simulink model "PCCI_Motor"  (R2023b)
settings: Solver=FixedStepDiscrete  StartTime=0.0  StopTime=10  FixedStep=0.01  RelTol=1e-3
settings Model: Creator=LENOVO-MCC  LastModifiedBy=LENOVO-MCC
settings OptimizationCC: DefaultParameterBehavior=Inlined  EnhancedBackFolding=on  PassReuseOutputArgsAs=Individual arguments  ZeroExternalMemoryAtStartup=off  ZeroInternalMemoryAtStartup=off  OptimizeBlockOrder=speed  DifferentSizesBufferReuse=on  OptimizationCustomize=off  EfficientTunableParamExpr=on
settings DebuggingCC: ParameterTunabilityLossMsg=error
settings SFSimCC: MATLABDynamicMemAlloc=off
settings RTWCC: Description=Embedded Coder  SystemTargetFile=ert.tlc  GenCodeOnly=on  TemplateMakefile=ert_default_tmf  GenerateReport=on  LaunchReport=on  GenerateCodeMetricsReport=on
settings CodeAppCC: ForceParamTrailComments=on  IgnoreCustomStorageClasses=off  OperatorAnnotations=on  SimulinkDataObjDesc=on  SFDataObjDesc=on  InsertBlockDesc=on
settings ERTTargetCC: TargetLangStandard=C99 (ISO)  GenerateSampleERTMain=on  InlinedParameterPlacement=NonHierarchical  ERTCustomFileTemplate=example_file_process.tlc

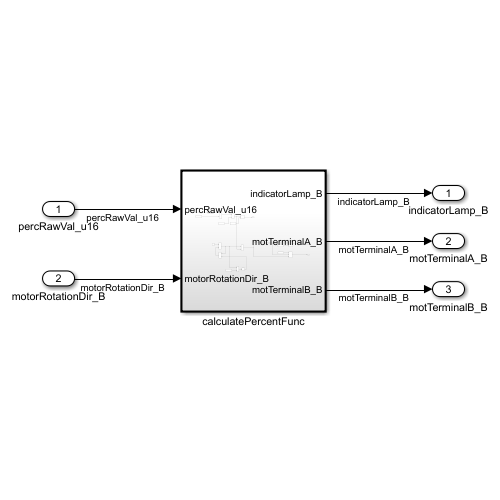
[thumbnail: Simulink's stored preview of the top-level diagram]
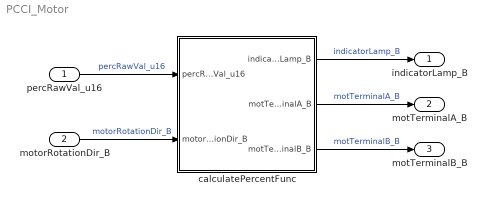
== system PCCI_Motor ==
  percRawVal_u16 : Inport  OutDataTypeStr=uint16
  motorRotationDir_B : Inport  Port=2  OutDataTypeStr=boolean
  calculatePercentFunc : Subsystem  TreatAsAtomicUnit=on
      settings: RTWFcnNameOpts=Use subsystem name  RTWFileNameOpts=Use subsystem name
  indicatorLamp_B : Outport  OutDataTypeStr=boolean
  motTerminalA_B : Outport  Port=2  OutDataTypeStr=boolean
  motTerminalB_B : Outport  Port=3  OutDataTypeStr=boolean
  wires:
  calculatePercentFunc/1(indicatorLamp_B) -> indicatorLamp_B/1  "indicatorLamp_B"
  percRawVal_u16/1 -> calculatePercentFunc/1(percRawVal_u16)  "percRawVal_u16"
  calculatePercentFunc/2(motTerminalA_B) -> motTerminalA_B/1  "motTerminalA_B"
  calculatePercentFunc/3(motTerminalB_B) -> motTerminalB_B/1  "motTerminalB_B"
  motorRotationDir_B/1 -> calculatePercentFunc/2(motorRotationDir_B)  "motorRotationDir_B"

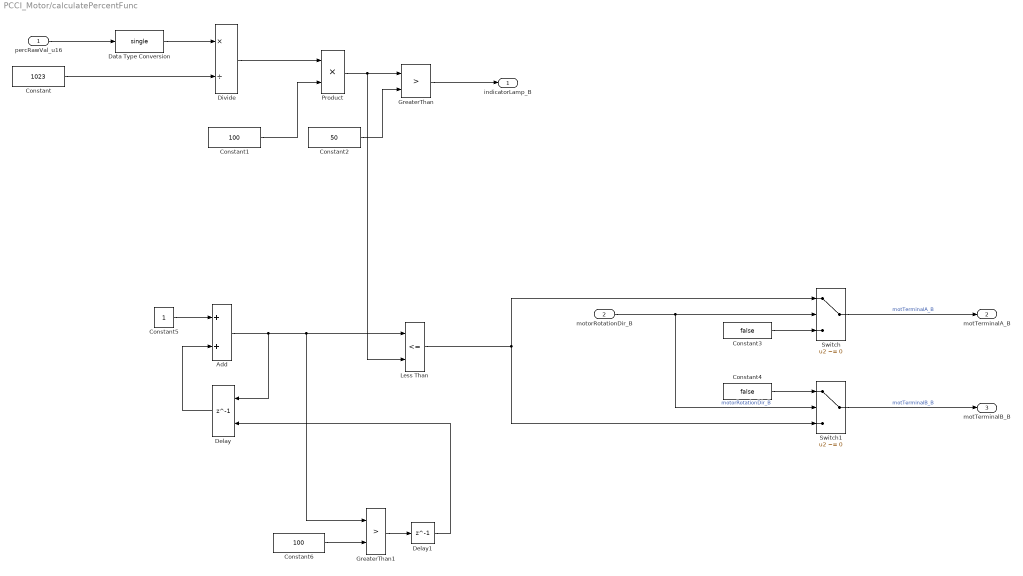
== system PCCI_Motor/calculatePercentFunc ==
  percRawVal_u16 : Inport  OutDataTypeStr=uint16
  motorRotationDir_B : Inport  Port=2  OutDataTypeStr=boolean
  Add : Sum
  Constant : Constant  Value=1023  OutDataTypeStr=single
  Constant1 : Constant  Value=100  OutDataTypeStr=int8
  Constant2 : Constant  Value=50  OutDataTypeStr=int8
  Constant3 : Constant  Value=false  OutDataTypeStr=boolean
  Constant4 : Constant  Value=false  OutDataTypeStr=boolean
  Constant5 : Constant  OutDataTypeStr=int8
  Constant6 : Constant  Value=100  OutDataTypeStr=int8
  Data Type Conversion : DataTypeConversion  OutDataTypeStr=single  SaturateOnIntegerOverflow=off  RndMeth=Floor
  Delay : Delay  DelayLength=1  ExternalReset=Rising
      settings: InputPortMap=u0,r5
  Delay1 : Delay  DelayLength=1
  Divide : Product  Inputs=*/
  GreaterThan : RelationalOperator  Operator=>  OutDataTypeStr=boolean  RndMeth=Simplest  InputSameDT=off
  GreaterThan1 : RelationalOperator  Operator=>  OutDataTypeStr=boolean  RndMeth=Simplest  InputSameDT=off
  Less Than : RelationalOperator  Operator=<=  OutDataTypeStr=boolean  RndMeth=Simplest  InputSameDT=off
  Product : Product
  Switch : Switch  Criteria=u2 ~= 0  SaturateOnIntegerOverflow=off  InputSameDT=off
  Switch1 : Switch  Criteria=u2 ~= 0  SaturateOnIntegerOverflow=off  InputSameDT=off
  indicatorLamp_B : Outport  OutDataTypeStr=boolean
  motTerminalA_B : Outport  Port=2  OutDataTypeStr=boolean
  motTerminalB_B : Outport  Port=3  OutDataTypeStr=boolean
  wires:
  percRawVal_u16/1 -> Data Type Conversion/1
  Data Type Conversion/1 -> Divide/1
  Constant/1 -> Divide/2
  Divide/1 -> Product/1
  Constant1/1 -> Product/2
  Constant2/1 -> GreaterThan/2
  GreaterThan/1 -> indicatorLamp_B/1
  Switch/1 -> motTerminalA_B/1  "motTerminalA_B"
  Switch1/1 -> motTerminalB_B/1  "motTerminalB_B"
  motorRotationDir_B/1 -> Switch1/2, Switch/2  "motorRotationDir_B"
  Constant3/1 -> Switch/3
  Constant4/1 -> Switch1/1
  Constant5/1 -> Add/1
  Add/1 -> Delay/1, GreaterThan1/1, Less Than/1
  Delay/1 -> Add/2
  Less Than/1 -> Switch1/3, Switch/1
  Constant6/1 -> GreaterThan1/2
  GreaterThan1/1 -> Delay1/1
  Delay1/1 -> Delay/2
  Product/1 -> Less Than/2, GreaterThan/1
